simulink model "closed_loop"  (R2020b)
settings: Solver=VariableStepAuto  StartTime=0.0  StopTime=10.0  RelTol=1e-3
settings Model: DataDictionary=closed_loop.sldd  Creator=ravenst1  LastModifiedBy=ravenst1

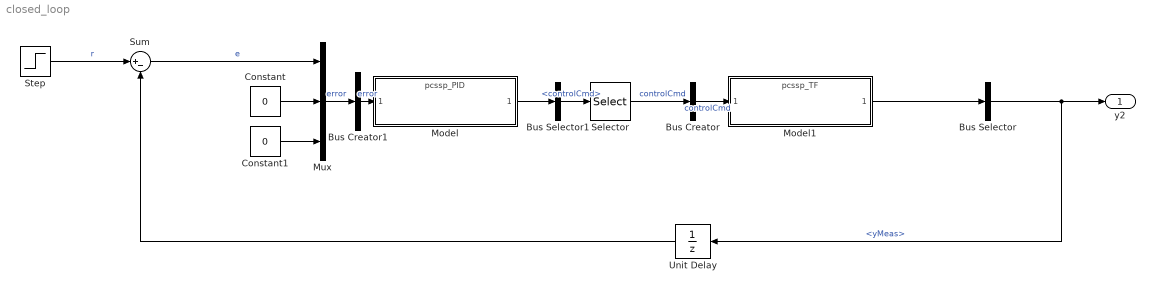
== system closed_loop ==
  Bus Creator : BusCreator  Inputs=1
  Bus Creator1 : BusCreator  Inputs=1  OutDataTypeStr=Bus: pcssp_PID_inBus
  Bus Selector : BusSelector  OutputSignals=yMeas
  Bus Selector1 : BusSelector  OutputSignals=controlCmd
  Constant : Constant  Value=0
  Constant1 : Constant  Value=0
  Model : ModelReference  ModelNameDialog=pcssp_PID.slx  UsingDefaultArgumentValue=0  SimulationMode=Normal  ModelReferenceVersion=1.19  tp=pcssp_PID_tp  SimulationMode=Normal
  Model1 : ModelReference  ModelNameDialog=pcssp_TF.slx  SimulationMode=Normal  ModelReferenceVersion=1.14
  Mux : Mux  Inputs=3
  Selector : Selector  InputPortWidth=3  IndexOptions=Index vector (dialog)  Indices=1  OutputSizes=1
  Step : Step  Time=2  SampleTime=0
  Sum : Sum  Inputs=|+-
  Unit Delay : UnitDelay  SampleTime=-1  HasFrameUpgradeWarning=on
  y2 : Outport
  wires:
  Model1/1 -> Bus Selector/1
  Step/1 -> Sum/1  "r"
  Unit Delay/1 -> Sum/2
  Sum/1 -> Mux/1  "e"
  Mux/1 -> Bus Creator1/1  "error"
  Selector/1 -> Bus Creator/1  "controlCmd"
  Bus Selector1/1 -> Selector/1  "<controlCmd>"
  Bus Creator1/1 -> Model/1  "error"
  Constant1/1 -> Mux/3
  Model/1 -> Bus Selector1/1
  Bus Selector/1 -> Unit Delay/1, y2/1  "<yMeas>"
  Constant/1 -> Mux/2
  Bus Creator/1 -> Model1/1  "controlCmd"
